simulink model "model_zbiorniki"  (R2015a)
settings: Solver=ode45  StartTime=0.0  StopTime=200  RelTol=1e-3
undefined symbols (not defined in the file or in its folder): alpha1, alpha2, alpha3, c1, c2, c3
settings Model: Creator=Student  LastModifiedBy=Student

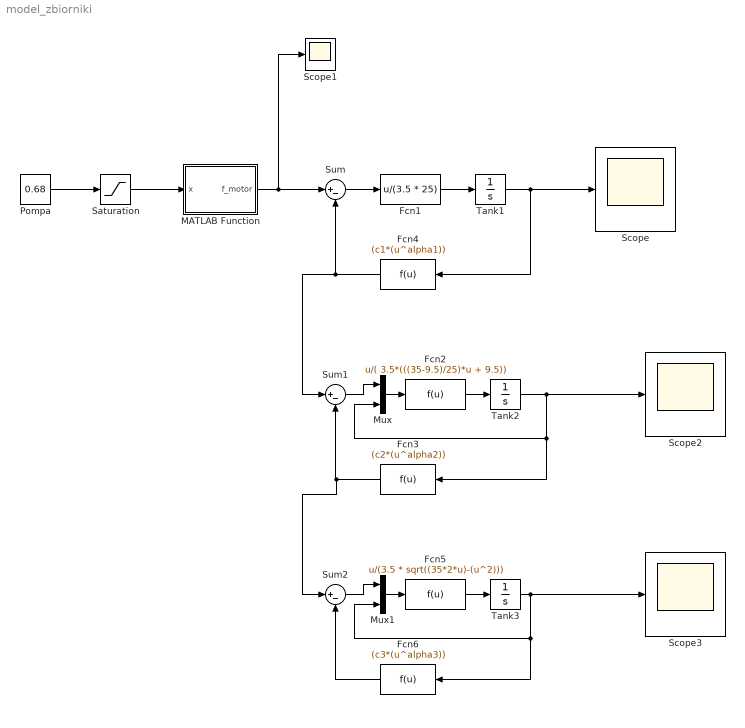
== system model_zbiorniki ==
  Fcn1 : Fcn  Expr=u/(3.5 * 25)
  Fcn2 : Fcn  Expr=u/( 3.5*(((35-9.5)/25)*u + 9.5))
  Fcn3 : Fcn  Expr=(c2*(u^alpha2))
  Fcn4 : Fcn  Expr=(c1*(u^alpha1))
  Fcn5 : Fcn  Expr=u/(3.5 * sqrt((35*2*u)-(u^2)))
  Fcn6 : Fcn  Expr=(c3*(u^alpha3))
  MATLAB Function : MATLAB Function  TreatAsAtomicUnit=on
  Mux : Mux  Inputs=2
  Mux1 : Mux  Inputs=2
  Pompa : Constant  Value=0.68
  Saturation : Saturate  UpperLimit=1  LowerLimit=0.5
  Scope{,1..3} (4 alike) : Scope
      Scope2 settings: SaveName=ScopeData2
      Scope3 settings: SaveName=ScopeData3
  Sum : Sum  Inputs=|+-
  Sum1 : Sum  Inputs=|+-
  Sum2 : Sum  Inputs=|+-
  Tank1 : Integrator  InitialCondition=0.1  LimitOutput=on  LowerSaturationLimit=0.1
  Tank2 : Integrator  InitialCondition=0.1  LimitOutput=on  LowerSaturationLimit=0.1
  Tank3 : Integrator  InitialCondition=0.1  LimitOutput=on  LowerSaturationLimit=0.1
  wires:
  Saturation/1 -> MATLAB Function/1(x)
  Pompa/1 -> Saturation/1
  MATLAB Function/1(f_motor) -> Scope1/1, Sum/1
  Sum/1 -> Fcn1/1
  Fcn1/1 -> Tank1/1
  Tank1/1 -> Fcn4/1, Scope/1
  Fcn4/1 -> Sum1/1, Sum/2
  Fcn2/1 -> Tank2/1
  Tank2/1 -> Mux/2, Fcn3/1, Scope2/1
  Fcn3/1 -> Sum2/1, Sum1/2
  Mux/1 -> Fcn2/1
  Sum1/1 -> Mux/1
  Fcn5/1 -> Tank3/1
  Tank3/1 -> Scope3/1, Mux1/2, Fcn6/1
  Fcn6/1 -> Sum2/2
  Mux1/1 -> Fcn5/1
  Sum2/1 -> Mux1/1

== matlab function model_zbiorniki/MATLAB Function ==
  data: x input; f_motor output
function f_motor = fcn(x)

a1_motor = 4.336406289988628e+02;
a2_motor = -1.346640151767827e+03;
a3_motor = 1.555231837686545e+03;
a4_motor = -5.004734794411548e+02;

f_motor = a1_motor * x^3 + a2_motor * x^2 + a3_motor * x + a4_motor;
